simulink model "TwoCar"  (R2017a)
settings: Solver=VariableStepAuto  StartTime=0.0  StopTime=100.0  RelTol=1e-3
settings Model: Creator=Carapinha  LastModifiedBy=Carapinha

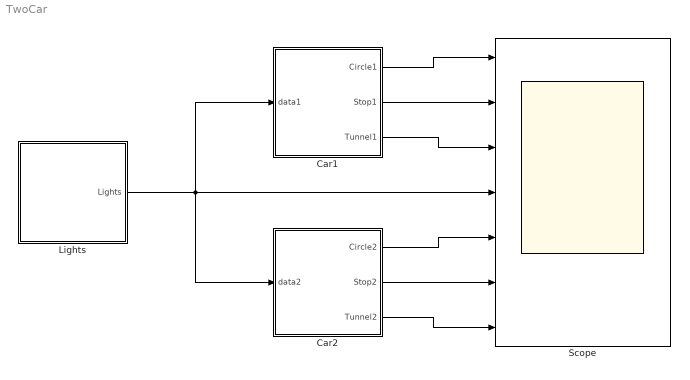
== system TwoCar ==
  Car1 : Stateflow chart  TreatAsAtomicUnit=on
  Car2 : Stateflow chart  TreatAsAtomicUnit=on
  Lights : Stateflow chart  TreatAsAtomicUnit=on
  Scope : Scope  NumInputPorts=7
  wires:
  Lights/1(Lights) -> Scope/4, Car2/1(data2), Car1/1(data1)
  Car2/3(Tunnel2) -> Scope/7
  Car2/1(Circle2) -> Scope/5
  Car2/2(Stop2) -> Scope/6
  Car1/1(Circle1) -> Scope/1
  Car1/2(Stop1) -> Scope/2
  Car1/3(Tunnel1) -> Scope/3

== stateflow chart TwoCar/Car1 ==
  state Tunnel
    entry:
    Circle1 = 0;
    Tunnel1 = 1;
    Stop1 = 0;
  state Lights
    entry:
    Circle1 = 0;
    Tunnel1 = 0;
    Stop1 = 1;
  state Circle
    entry:
    Circle1 = 1;
    Tunnel1 = 0;
    Stop1 = 0;
  (default) -> Lights
  Lights -> Tunnel [order 1] : [data1 == 1]
  Lights -> Lights [order 2] : [data1 == 0 || data1 == -1]
  Circle -> Lights : [after(3,sec)]
  Tunnel -> Circle : [after(3,sec)]
  data: data1 input; Circle1 output; Stop1 output; Tunnel1 output

== stateflow chart TwoCar/Car2 ==
  state Tunnel3
    entry:
    Circle2 = 0;
    Tunnel2 = 1;
    Stop2 = 0;
  state Lights3
    entry:
    Circle2 = 0;
    Tunnel2 = 0;
    Stop2 = 1;
  state Circle3
    entry:
    Circle2 = 1;
    Tunnel2 = 0;
    Stop2 = 0;
  (default) -> Lights3
  Lights3 -> Tunnel3 [order 1] : [data2 == -1]
  Lights3 -> Lights3 [order 2] : [data2 == 0 || data2 == 1]
  Circle3 -> Lights3 : [after(3,sec)]
  Tunnel3 -> Circle3 : [after(3,sec)]
  data: data2 input; Circle2 output; Stop2 output; Tunnel2 output

== stateflow chart TwoCar/Lights ==
  state RR
    entry:
    Lights = 0;
  state RG
    entry:
    Lights = -1;
  state GR
    entry:
    Lights = 1;
  (default) -> RR
  RR -> RG : [after(10,sec)]
  GR -> RR : [after(10,sec)]
  RG -> GR : [after(10,sec)]
  data: Lights output
